simulink model "modelo_SIRV"  (R2019b)
settings: Solver=VariableStepAuto  StartTime=0.0  StopTime=30  RelTol=1e-3
settings Model: Creator=lucia  LastModifiedBy=lucia

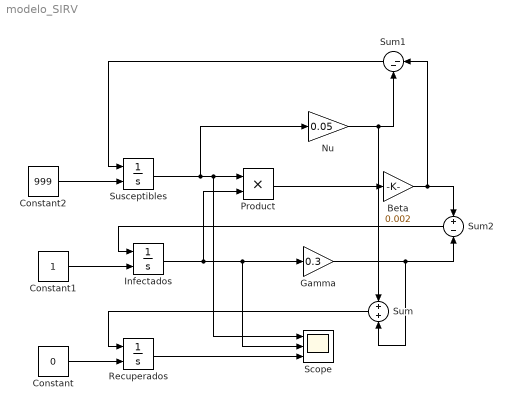
== system modelo_SIRV ==
  Beta : Gain  Gain=0.002
  Constant : Constant  Value=0
  Constant1 : Constant
  Constant2 : Constant  Value=999
  Gamma : Gain  Gain=0.3
  Infectados : Integrator  InitialConditionSource=external
  Nu : Gain  Gain=0.05
  Product : Product
  Recuperados : Integrator  InitialConditionSource=external
  Scope : Scope  NumInputPorts=3
  Sum : Sum
  Sum1 : Sum  Inputs=|--
  Sum2 : Sum  Inputs=+-
  Susceptibles : Integrator  InitialConditionSource=external
  wires:
  Infectados/1 -> Product/2, Scope/2, Gamma/1
  Product/1 -> Beta/1
  Susceptibles/1 -> Scope/1, Product/1, Nu/1
  Constant1/1 -> Infectados/2
  Constant2/1 -> Susceptibles/2
  Beta/1 -> Sum1/1, Sum2/1
  Nu/1 -> Sum1/2, Sum/1
  Sum1/1 -> Susceptibles/1
  Gamma/1 -> Sum/2, Sum2/2
  Sum2/1 -> Infectados/1
  Constant/1 -> Recuperados/2
  Sum/1 -> Recuperados/1
  Recuperados/1 -> Scope/3
